simulink subsystem "Day4_5_Scenario_1"  (R2024a)
settings: Solver=VariableStepAuto  StartTime=0.0  StopTime=10.0  RelTol=1e-3
libraries: CarMaker4SL x44
(part 5 of 5)

== matlab function Day4_5_Scenario_1/MATLAB Function ==
  data: map input size=[100 100]; path output size=[30 4]; start_point input size=[2 1]; finish_point input size=[2 1]; goal_yaw input
function path = path_planner_(map, start_point, finish_point, goal_yaw)
persistent cached_path cached_sx cached_sy cached_gx cached_gy cached_yaw cached_count cached_rsum cached_csum cached_ready

N = 30;
MAP_N = 100;
NX = 45;
NY = 45;
NYAW = 16;
MAX_NODE = 7000;
MAX_ITER = 7000;
PI = 3.141592653589793;

path = zeros(N, 4);

sx = start_point(1);
sy = start_point(2);
gx = finish_point(1);
gy = finish_point(2);

while goal_yaw > PI
    goal_yaw = goal_yaw - 2 * PI;
end
while goal_yaw < -PI
    goal_yaw = goal_yaw + 2 * PI;
end

map_count = 0;
map_rsum = 0;
map_csum = 0;
for r = 1:MAP_N
    for c = 1:MAP_N
        if map(r, c) > 0.5
            map_count = map_count + 1;
            map_rsum = map_rsum + r;
            map_csum = map_csum + c;
        end
    end
end

if isempty(cached_ready)
    cached_ready = 0;
    cached_path = path;
    cached_sx = 9999;
    cached_sy = 9999;
    cached_gx = 9999;
    cached_gy = 9999;
    cached_yaw = 9999;
    cached_count = -1;
    cached_rsum = -1;
    cached_csum = -1;
end

if cached_ready == 1
    if abs(cached_sx - sx) < 0.05 && abs(cached_sy - sy) < 0.05 && ...
       abs(cached_gx - gx) < 0.05 && abs(cached_gy - gy) < 0.05 && ...
       abs(cached_yaw - goal_yaw) < 0.01 && ...
       cached_count == map_count && cached_rsum == map_rsum && cached_csum == map_csum
        path = cached_path;
        return;
    end
end

x_min = 0.0;
x_max = 100.0;
y_min = -100.0;
y_max = 0.0;

start_yaw = atan2(gy - sy, gx - sx);
while start_yaw > PI
    start_yaw = start_yaw - 2 * PI;
end
while start_yaw < -PI
    start_yaw = start_yaw + 2 * PI;
end

node_x = zeros(MAX_NODE, 1);
node_y = zeros(MAX_NODE, 1);
node_yaw = zeros(MAX_NODE, 1);
node_g = zeros(MAX_NODE, 1);
node_parent = zeros(MAX_NODE, 1);
node_dir = ones(MAX_NODE, 1);

open_list = zeros(MAX_NODE, 1);
g_best = 1.0e9 * ones(NY, NX, NYAW);
best_node = zeros(NY, NX, NYAW);
closed = zeros(NY, NX, NYAW);

node_count = 1;
open_count = 1;

node_x(1) = sx;
node_y(1) = sy;
node_yaw(1) = start_yaw;
node_g(1) = 0;
node_parent(1) = 0;
node_dir(1) = 1;
open_list(1) = 1;

ix = round((sx - x_min) / (x_max - x_min) * (NX - 1)) + 1;
iy = round((sy - y_min) / (y_max - y_min) * (NY - 1)) + 1;
iyaw = round((start_yaw + PI) / (2 * PI) * (NYAW - 1)) + 1;
ix = min(max(ix, 1), NX);
iy = min(max(iy, 1), NY);
iyaw = min(max(iyaw, 1), NYAW);
g_best(iy, ix, iyaw) = 0;
best_node(iy, ix, iyaw) = 1;

steer_list = [-0.55, -0.28, 0.0, 0.28, 0.55];
dir_list = [1, -1];
step = 3.0;
wheel_base = 2.7;

goal_node = 1;
found = 0;
best_goal_score = 1.0e9;

for iter = 1:MAX_ITER
    if open_count <= 0
        break;
    end

    best_open_pos = 1;
    best_f = 1.0e9;

    for oi = 1:MAX_NODE
        if oi > open_count
            break;
        end

        nid = open_list(oi);

        dxg = gx - node_x(nid);
        dyg = gy - node_y(nid);
        dist_h = sqrt(dxg * dxg + dyg * dyg);

        yaw_err = goal_yaw - node_yaw(nid);
        while yaw_err > PI
            yaw_err = yaw_err - 2 * PI;
        end
        while yaw_err < -PI
            yaw_err = yaw_err + 2 * PI;
        end

        f = node_g(nid) + dist_h + 1.5 * abs(yaw_err);

        if f < best_f
            best_f = f;
            best_open_pos = oi;
        end
    end

    cur = open_list(best_open_pos);
    open_list(best_open_pos) = open_list(open_count);
    open_list(open_count) = 0;
    open_count = open_count - 1;

    ix = round((node_x(cur) - x_min) / (x_max - x_min) * (NX - 1)) + 1;
    iy = round((node_y(cur) - y_min) / (y_max - y_min) * (NY - 1)) + 1;
    iyaw = round((node_yaw(cur) + PI) / (2 * PI) * (NYAW - 1)) + 1;
    ix = min(max(ix, 1), NX);
    iy = min(max(iy, 1), NY);
    iyaw = min(max(iyaw, 1), NYAW);

    if closed(iy, ix, iyaw) == 1
        continue;
    end

    closed(iy, ix, iyaw) = 1;

    dxg = gx - node_x(cur);
    dyg = gy - node_y(cur);
    goal_dist = sqrt(dxg * dxg + dyg * dyg);

    yaw_err = goal_yaw - node_yaw(cur);
    while yaw_err > PI
        yaw_err = yaw_err - 2 * PI;
    end
    while yaw_err < -PI
        yaw_err = yaw_err + 2 * PI;
    end

    goal_score = goal_dist + 2.0 * abs(yaw_err);
    if goal_score < best_goal_score
        best_goal_score = goal_score;
        goal_node = cur;
    end

    if goal_dist < 3.0 && abs(yaw_err) < 0.8
        goal_node = cur;
        found = 1;
        break;
    end

    for di = 1:2
        move_dir = dir_list(di);

        for si = 1:5
            steer = steer_list(si);

            new_x = node_x(cur) + move_dir * step * cos(node_yaw(cur));
            new_y = node_y(cur) + move_dir * step * sin(node_yaw(cur));
            new_yaw = node_yaw(cur) + move_dir * step / wheel_base * tan(steer);

            while new_yaw > PI
                new_yaw = new_yaw - 2 * PI;
            end
            while new_yaw < -PI
                new_yaw = new_yaw + 2 * PI;
            end

            if new_x < x_min || new_x > x_max || new_y < y_min || new_y > y_max
                continue;
            end

            valid = 1;

            for samp = 1:6
                a = samp / 6.0;
                px = node_x(cur) * (1 - a) + new_x * a;
                py = node_y(cur) * (1 - a) + new_y * a;

                mr = round((py - y_min) / (y_max - y_min) * (MAP_N - 1)) + 1;
                mc = round((px - x_min) / (x_max - x_min) * (MAP_N - 1)) + 1;

                if mr < 1 || mr > MAP_N || mc < 1 || mc > MAP_N
                    valid = 0;
                else
                    for rr = -1:1
                        for cc = -1:1
                            r2 = min(max(mr + rr, 1), MAP_N);
                            c2 = min(max(mc + cc, 1), MAP_N);

                            if map(r2, c2) > 0.5
                                valid = 0;
                            end
                        end
                    end
                end
            end

            if valid == 0
                continue;
            end

            nix = round((new_x - x_min) / (x_max - x_min) * (NX - 1)) + 1;
            niy = round((new_y - y_min) / (y_max - y_min) * (NY - 1)) + 1;
            niyaw = round((new_yaw + PI) / (2 * PI) * (NYAW - 1)) + 1;

            nix = min(max(nix, 1), NX);
            niy = min(max(niy, 1), NY);
            niyaw = min(max(niyaw, 1), NYAW);

            if closed(niy, nix, niyaw) == 1
                continue;
            end

            move_cost = step;
            if move_dir < 0
                move_cost = move_cost + 1.0;
            end
            move_cost = move_cost + 0.6 * abs(steer);

            if move_dir ~= node_dir(cur)
                move_cost = move_cost + 4.0;
            end

            new_g = node_g(cur) + move_cost;

            if new_g < g_best(niy, nix, niyaw)
                if node_count < MAX_NODE && open_count < MAX_NODE
                    node_count = node_count + 1;
                    nid2 = node_count;

                    node_x(nid2) = new_x;
                    node_y(nid2) = new_y;
                    node_yaw(nid2) = new_yaw;
                    node_g(nid2) = new_g;
                    node_parent(nid2) = cur;
                    node_dir(nid2) = move_dir;

                    g_best(niy, nix, niyaw) = new_g;
                    best_node(niy, nix, niyaw) = nid2;

                    open_count = open_count + 1;
                    open_list(open_count) = nid2;
                end
            end
        end
    end
end

temp_id = zeros(MAX_NODE, 1);
temp_len = 0;
cur = goal_node;

for k = 1:MAX_NODE
    if cur <= 0
        break;
    end

    temp_len = temp_len + 1;
    temp_id(temp_len) = cur;

    if cur == 1
        break;
    end

    cur = node_parent(cur);
end

if temp_len > 1
    for i = 1:N
        a = (i - 1) / (N - 1);
        tidx = round(temp_len - a * (temp_len - 1));
        tidx = min(max(tidx, 1), temp_len);
        nid = temp_id(tidx);

        path(i, 1) = node_x(nid);
        path(i, 2) = node_y(nid);
        path(i, 3) = node_yaw(nid);
        path(i, 4) = node_dir(nid);
    end
else
    wp = zeros(5, 2);
    wp(1, 1) = sx;
    wp(1, 2) = sy;
    wp(2, 1) = 24.0;
    wp(2, 2) = -62.0;
    wp(3, 1) = 86.0;
    wp(3, 2) = -62.0;
    wp(4, 1) = 86.0;
    wp(4, 2) = gy;
    wp(5, 1) = gx;
    wp(5, 2) = gy;

    for i = 1:N
        a = (i - 1) / (N - 1);
        seg_float = a * 4.0;
        seg = floor(seg_float) + 1;

        if seg >= 5
            seg = 4;
            local_a = 1.0;
        else
            local_a = seg_float - floor(seg_float);
        end

        path(i, 1) = wp(seg, 1) * (1 - local_a) + wp(seg + 1, 1) * local_a;
        path(i, 2) = wp(seg, 2) * (1 - local_a) + wp(seg + 1, 2) * local_a;
        path(i, 4) = 1;
    end
end

path(1, 1) = sx;
path(1, 2) = sy;
path(N, 1) = gx;
path(N, 2) = gy;
path(N, 3) = goal_yaw;

for i = 1:N-1
    dx = path(i + 1, 1) - path(i, 1);
    dy = path(i + 1, 2) - path(i, 2);

    if sqrt(dx * dx + dy * dy) > 0.01
        if path(i, 4) >= 0
            path(i, 3) = atan2(dy, dx);
        else
            path(i, 3) = atan2(dy, dx) + PI;
            while path(i, 3) > PI
                path(i, 3) = path(i, 3) - 2 * PI;
            end
        end
    end

    if path(i, 4) >= 0
        path(i, 4) = 1;
    else
        path(i, 4) = -1;
    end
end

path(N, 4) = path(N - 1, 4);

cached_path = path;
cached_sx = sx;
cached_sy = sy;
cached_gx = gx;
cached_gy = gy;
cached_yaw = goal_yaw;
cached_count = map_count;
cached_rsum = map_rsum;
cached_csum = map_csum;
cached_ready = 1;
end

== matlab function Day4_5_Scenario_1/MATLAB Function4 ==
  data: ego_x input; desired_ax output; ego_y input; ego_vx input; tire_angle output; gear_cmd output; vc_gas output; vc_brake output
function [desired_ax, tire_angle, gear_cmd, vc_gas, vc_brake] = reverse_test_(ego_x, ego_y, ego_vx)
persistent phase start_x start_y reverse_x reverse_y stop_count

ego_x = ego_x(1);
ego_y = ego_y(1);
ego_vx = ego_vx(1);

tire_angle = 0;
desired_ax = 0;

if isempty(phase)
    phase = 1;
    start_x = ego_x;
    start_y = ego_y;
    reverse_x = ego_x;
    reverse_y = ego_y;
    stop_count = 0;
end

speed_abs = abs(ego_vx);

dx0 = ego_x - start_x;
dy0 = ego_y - start_y;
forward_dist = sqrt(dx0 * dx0 + dy0 * dy0);

dxr = ego_x - reverse_x;
dyr = ego_y - reverse_y;
reverse_dist = sqrt(dxr * dxr + dyr * dyr);

forward_target_dist = 20.0;
reverse_target_dist = 8.0;

gear_cmd = 1;
vc_gas = 0;
vc_brake = 0;

if phase == 1
    % 전진
    gear_cmd = 1;
    vc_gas = 0.12;
    vc_brake = 0;
    desired_ax = 0;

    if forward_dist > forward_target_dist
        phase = 2;
        stop_count = 0;
    end

elseif phase == 2
    % 전진 정지
    gear_cmd = 1;
    vc_gas = 0;
    vc_brake = 0.35;
    desired_ax = 0;

    if speed_abs < 0.15
        stop_count = stop_count + 1;
    else
        stop_count = 0;
    end

    if stop_count > 30
        phase = 3;
        reverse_x = ego_x;
        reverse_y = ego_y;
        stop_count = 0;
    end

elseif phase == 3
    % 후진
    gear_cmd = -1;
    vc_gas = 0.30;
    vc_brake = 0;
    desired_ax = 0;

    if reverse_dist > reverse_target_dist
        phase = 4;
        stop_count = 0;
    end

else
    % 후진 정지
    gear_cmd = -1;
    vc_gas = 0;
    vc_brake = 0.35;
    desired_ax = 0;
end

end
